simulink model "muscleLegs_task2"  (R2025b)
settings: Solver=ode23t  StartTime=0.0  StopTime=t_end  MaxStep=1e-3  RelTol=1e-4
values from neighbouring files (symbols this model uses):
  c = 0.05    [setup_muscleLegs_nm.m]
  CtrlPar = [tau_H_st; phi_K_tgt_st; P_K_st; D_K_st ... (first row only)    [setup_muscleLegs_ctrl.m]
  eref_se = 0.04    [setup_muscleLegs_nm.m]
  FmaxBFSH = 350    [setup_muscleLegs_nm.m]
  FmaxGLU = 4000    [setup_muscleLegs_nm.m]
  FmaxHFL = 2000    [setup_muscleLegs_nm.m]
  FmaxVAS = 5000    [setup_muscleLegs_nm.m]
  g = 9.81    [setup_muscleLegs_model.m]
  G_dtheta_GLU = 5    [setup_muscleLegs_ctrl.m]    (also in sim_muscleLegs_Task2.m = base_G_dtheta_GLU * optim_vals(15); sim_muscleLegs_Task3.m = base_G(2) * optim_vals(15))
  G_theta_GLU = 60    [setup_muscleLegs_ctrl.m]    (also in sim_muscleLegs_Task2.m = base_G_theta_GLU * optim_vals(14); sim_muscleLegs_Task3.m = base_G(1) * optim_vals(14))
  init_stim = 0.01    [setup_muscleLegs_nm.m]
  K = 5    [setup_muscleLegs_nm.m]
  l_HAT = 0.8    [setup_muscleLegs_model.m]
  l_shank = l_leg/2    (= 0.49)    [setup_muscleLegs_model.m]
  l_thigh = l_leg/2    (= 0.49)    [setup_muscleLegs_model.m]
  loptBFSH = 0.12    [setup_muscleLegs_nm.m]
  loptGLU = 0.11    [setup_muscleLegs_nm.m]
  loptHFL = 0.11    [setup_muscleLegs_nm.m]
  loptVAS = 0.08    [setup_muscleLegs_nm.m]
  lslackBFSH = 0.10    (= 0.1)    [setup_muscleLegs_nm.m]
  lslackGLU = 0.13    [setup_muscleLegs_nm.m]
  lslackHFL = 0.10    (= 0.1)    [setup_muscleLegs_nm.m]
  lslackVAS = 0.23    [setup_muscleLegs_nm.m]
  m_HAT = 54    [setup_muscleLegs_model.m]
  m_shank = 4    [setup_muscleLegs_model.m]
  m_thigh = 8    [setup_muscleLegs_model.m]
  N = 12    [cmaes_task1_2_set1.mat]    (also in cmaes_task1_2_set2.mat; cmaes_task2_2_set1.mat = 17; cmaes_task2_2_set2.mat = 17; cmaes_task3_crouch.mat = 17)
  phirefBFSH = 160*pi/180    (= 2.79252680319)    [setup_muscleLegs_nm.m]
  phirefGLU = 60*pi/180    (= 1.0471975512)    [setup_muscleLegs_nm.m]
  phirefHFL = 20*pi/180    (= 0.349065850399)    [setup_muscleLegs_nm.m]
  phirefVAS = 60*pi/180    (= 1.0471975512)    [setup_muscleLegs_nm.m]
  plane_height = 0.1    [setup_muscleLegs_model.m]
  plane_x = 100    [setup_muscleLegs_model.m]
  plane_z = 1    [setup_muscleLegs_model.m]
  r_foot = 0.01    [setup_muscleLegs_model.m]
  rBFSH = 0.04    [setup_muscleLegs_nm.m]
  rGLU = 0.08    [setup_muscleLegs_nm.m]
  rHFL = 0.08    [setup_muscleLegs_nm.m]
  rhoBFSH = 0.7    [setup_muscleLegs_nm.m]
  rhoGLU = 0.5    [setup_muscleLegs_nm.m]
  rhoHFL = 0.5    [setup_muscleLegs_nm.m]
  rhoVAS = 0.6    [setup_muscleLegs_nm.m]
  rVAS = 0.05    [setup_muscleLegs_nm.m]
  tau_act = 0.01    [setup_muscleLegs_nm.m]
  tau_deact = 0.04    [setup_muscleLegs_nm.m]
  theta_tgt = 0.001    [setup_muscleLegs_ctrl.m]    (also in sim_muscleLegs_Task2.m = 0 + (optim_vals(13) - 1) * 0.1; sim_muscleLegs_Task3.m = 0 + (optim_vals(13) - 1) * 0.1)
  vi_Ctrl_st = 1:4    [setup_muscleLegs_ctrl.m]
  vi_Ctrl_sw = 5:12    [setup_muscleLegs_ctrl.m]
  vmaxBFSH = 12    [setup_muscleLegs_nm.m]
  vmaxGLU = 12    [setup_muscleLegs_nm.m]
  vmaxHFL = 12    [setup_muscleLegs_nm.m]
  vmaxVAS = 12    [setup_muscleLegs_nm.m]
  w = 0.56    [setup_muscleLegs_nm.m]
  w_pe = w    (= 0.56)    [setup_muscleLegs_nm.m]
undefined symbols (not defined in the file or in its folder): l1, X, Y, Z
libraries: sm_lib x30, nesl_utility x19, simulink x1
(part 3 of 4)

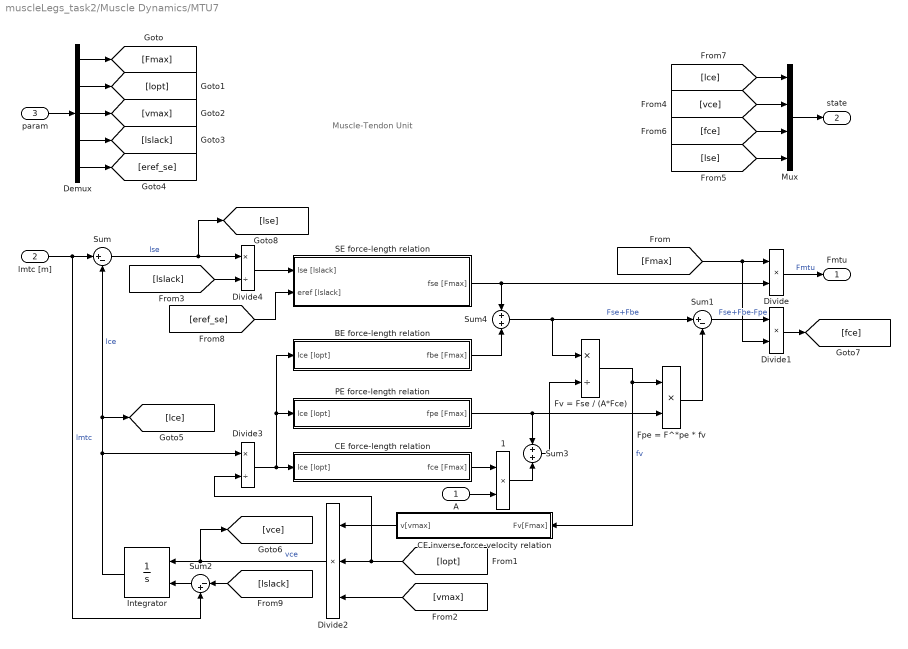
== system muscleLegs_task2/Muscle Dynamics/MTU7 ==
  note: Muscle-Tendon Unit
  A : Inport
  lmtc [m] : Inport  Port=2
  param : Inport  Port=3
  1 : Product  Inputs=**  InputSameDT=on  SaturateOnIntegerOverflow=on  OutDataTypeStr=Inherit: Same as first input
  BE force-length relation : Subsystem
  CE force-length relation : Subsystem
  CE inverse force-velocity relation : Subsystem
  Demux : Demux  Outputs=5
  Divide : Product
  Divide1 : Product
  Divide2 : Product  Inputs=3
  Divide3 : Product  Inputs=*/
  Divide4 : Product  Inputs=*/
  "Fpe = F^*pe * fv " : Product  InputSameDT=on  SaturateOnIntegerOverflow=on  OutDataTypeStr=Inherit: Same as first input
  Fv = Fse / (A*Fce) : Product  Inputs=*/  InputSameDT=on  SaturateOnIntegerOverflow=on  OutDataTypeStr=Inherit: Same as first input
  Integrator : Integrator  InitialConditionSource=external  LowerSaturationLimit=0.05
  Mux : Mux
  PE force-length relation : Subsystem
  SE force-length relation : Subsystem
  Sum : Sum  Inputs=|+-  InputSameDT=on  SaturateOnIntegerOverflow=on  OutDataTypeStr=Inherit: Same as first input
  Sum1 : Sum  Inputs=|+-  InputSameDT=on  SaturateOnIntegerOverflow=on  OutDataTypeStr=Inherit: Same as first input
  Sum2 : Sum  Inputs=|-+  InputSameDT=on  SaturateOnIntegerOverflow=on  OutDataTypeStr=Inherit: Same as first input
  Sum3 : Sum  InputSameDT=on  SaturateOnIntegerOverflow=on  OutDataTypeStr=Inherit: Same as first input
  Sum4 : Sum  InputSameDT=on  SaturateOnIntegerOverflow=on  OutDataTypeStr=Inherit: Same as first input
  Fmtu : Outport  InitialOutput=0  VectorParamsAs1DForOutWhenUnconnected=off
  state : Outport  Port=2  InitialOutput=0  VectorParamsAs1DForOutWhenUnconnected=off
  wires:
  Integrator/1 -> Divide3/1, [lce], Sum/2  "lce"
  Divide3/1 -> CE force-length relation/1(lce [lopt]), PE force-length relation/1(lce [lopt]), BE force-length relation/1(lce [lopt])
  Fv = Fse / (A*Fce)/1 -> CE inverse force-velocity relation/1(Fv[Fmax]), "Fpe = F^*pe * fv "/1  "fv"
  Divide2/1 -> [vce], Integrator/1  "vce"
  lmtc [m]/1 -> Sum/1, Sum2/2  "lmtc"
  Divide/1 -> Fmtu/1  "Fmtu"
  Divide4/1 -> SE force-length relation/1(lse [lslack])
  SE force-length relation/1(fse [Fmax]) -> Sum4/1, Divide/2
  Sum2/1 -> Integrator/2
  [lslack] -> Sum2/1
  CE force-length relation/1(fce [Fmax]) -> 1/1
  PE force-length relation/1(fpe [Fmax]) -> "Fpe = F^*pe * fv "/2, Sum3/1
  1/1 -> Sum3/2
  BE force-length relation/1(fbe [Fmax]) -> Sum4/2
  Sum3/1 -> Fv = Fse / (A*Fce)/2
  CE inverse force-velocity relation/1(v[vmax]) -> Divide2/1
  A/1 -> 1/2
  Sum4/1 -> Sum1/1, Fv = Fse / (A*Fce)/1  "Fse+Fbe"
  "Fpe = F^*pe * fv "/1 -> Sum1/2
  Sum1/1 -> Divide1/1  "Fse+Fbe-Fpe"
  Divide1/1 -> [fce]
  Sum/1 -> [lse], Divide4/1  "lse"
  [lopt] -> Divide2/2, Divide3/2
  [vmax] -> Divide2/3
  [lslack] -> Divide4/2
  param/1 -> Demux/1
  Demux/1 -> [Fmax]
  Demux/2 -> [lopt]
  Demux/4 -> [lslack]
  Demux/3 -> [vmax]
  Demux/5 -> [eref_se]
  [Fmax] -> Divide1/2, Divide/1
  Mux/1 -> state/1
  [lce] -> Mux/1
  [vce] -> Mux/2
  [fce] -> Mux/3
  [lse] -> Mux/4
  [eref_se] -> SE force-length relation/2(eref [lslack])

== system muscleLegs_task2/Neural Control/Stance L ==
  CtrlPar : Inport
  phi_K : Inport  Port=2
  d_phi_K : Inport  Port=3
  d_theta : Inport  Port=4
  theta : Inport  Port=5
  d_theta1 : Inport  Port=6
  theta1 : Inport  Port=7
  Enable : EnablePort
  Constant : Constant  Value=theta_tgt
  Constant1 : Constant  Value=theta_tgt
  Constant2 : Constant  Value=0
  Demux : Demux  Outputs=length(vi_Ctrl_st)
  Divide : Product
  Divide1 : Product
  Gain : Gain  Gain=-1
  Gain1 : Gain  Gain=G_theta_GLU
  Gain2 : Gain  Gain=G_dtheta_GLU
  Gain3 : Gain  Gain=-G_theta_GLU
  Gain4 : Gain  Gain=-G_dtheta_GLU
  Sum{,1,5..6} (4 alike) : Sum  Inputs=|+-
  Sum2 : Sum  Inputs=|++
  Sum3 : Sum  Inputs=|++
  Sum4 : Sum  Inputs=|++
  extension : Saturate  UpperLimit=1  LowerLimit=0.01
  extension1 : Saturate  UpperLimit=1  LowerLimit=0.01
  flexion : Saturate  UpperLimit=1  LowerLimit=0.01
  flexion1 : Saturate  UpperLimit=1  LowerLimit=0.01
  S_VAS : Outport  OutputWhenDisabled=reset  InitialOutput=0
  S_BFSH : Outport  Port=2  OutputWhenDisabled=reset  InitialOutput=0
  S_GLU : Outport  Port=3  OutputWhenDisabled=reset  InitialOutput=0
  S_HFL : Outport  Port=4  OutputWhenDisabled=reset  InitialOutput=0
  wires:
  Divide1/1 -> Sum2/2
  d_phi_K/1 -> Sum1/2
  phi_K/1 -> Sum/2
  Divide/1 -> Sum2/1
  Sum/1 -> Divide/2
  Sum1/1 -> Divide1/2
  Constant2/1 -> Sum1/1
  CtrlPar/1 -> Demux/1
  Demux/2 -> Sum/1  "phi_K_tgt_st"
  Demux/3 -> Divide/1  "P_K_st"
  Demux/4 -> Divide1/1  "D_K_st"
  extension/1 -> S_VAS/1
  Gain/1 -> extension/1
  Sum2/1 -> flexion/1, Gain/1
  flexion/1 -> S_BFSH/1
  Sum3/1 -> extension1/1
  extension1/1 -> S_GLU/1
  flexion1/1 -> S_HFL/1
  Gain1/1 -> Sum3/1
  Gain2/1 -> Sum3/2
  d_theta/1 -> Gain2/1
  d_theta1/1 -> Gain4/1
  Sum4/1 -> flexion1/1
  Gain4/1 -> Sum4/2
  Gain3/1 -> Sum4/1
  theta/1 -> Sum5/1
  Sum5/1 -> Gain1/1
  Constant/1 -> Sum5/2
  theta1/1 -> Sum6/1
  Sum6/1 -> Gain3/1
  Constant1/1 -> Sum6/2

== system muscleLegs_task2/Neural Control/Stance R ==
  CtrlPar : Inport
  phi_K : Inport  Port=2
  d_phi_K : Inport  Port=3
  d_theta1 : Inport  Port=4
  theta1 : Inport  Port=5
  d_theta2 : Inport  Port=6
  theta2 : Inport  Port=7
  Enable : EnablePort
  Constant : Constant  Value=theta_tgt
  Constant1 : Constant  Value=theta_tgt
  Constant2 : Constant  Value=0
  Demux : Demux  Outputs=length(vi_Ctrl_st)
  Divide : Product
  Divide1 : Product
  Gain : Gain  Gain=-1
  Gain1 : Gain  Gain=G_theta_GLU
  Gain2 : Gain  Gain=G_dtheta_GLU
  Gain3 : Gain  Gain=-G_theta_GLU
  Gain4 : Gain  Gain=-G_dtheta_GLU
  Sum{,1,5..6} (4 alike) : Sum  Inputs=|+-
  Sum2 : Sum  Inputs=|++
  Sum3 : Sum  Inputs=|++
  Sum4 : Sum  Inputs=|++
  extension : Saturate  UpperLimit=1  LowerLimit=0.01
  extension1 : Saturate  UpperLimit=1  LowerLimit=0.01
  flexion : Saturate  UpperLimit=1  LowerLimit=0.01
  flexion1 : Saturate  UpperLimit=1  LowerLimit=0.01
  S_VAS : Outport  OutputWhenDisabled=reset  InitialOutput=0
  S_BFSH : Outport  Port=2  OutputWhenDisabled=reset  InitialOutput=0
  S_GLU : Outport  Port=3  OutputWhenDisabled=reset  InitialOutput=0
  S_HFL : Outport  Port=4  OutputWhenDisabled=reset  InitialOutput=0
  wires:
  Divide1/1 -> Sum2/2
  d_phi_K/1 -> Sum1/2
  phi_K/1 -> Sum/2
  Divide/1 -> Sum2/1
  Sum/1 -> Divide/2
  Sum1/1 -> Divide1/2
  Constant2/1 -> Sum1/1
  CtrlPar/1 -> Demux/1
  Demux/2 -> Sum/1  "phi_K_tgt_st"
  Demux/3 -> Divide/1  "P_K_st"
  Demux/4 -> Divide1/1  "D_K_st"
  flexion/1 -> S_BFSH/1
  Sum2/1 -> flexion/1, Gain/1
  extension/1 -> S_VAS/1
  Gain/1 -> extension/1
  Sum4/1 -> flexion1/1
  Gain3/1 -> Sum4/1
  Gain4/1 -> Sum4/2
  d_theta2/1 -> Gain4/1
  Sum3/1 -> extension1/1
  Gain2/1 -> Sum3/2
  extension1/1 -> S_GLU/1
  flexion1/1 -> S_HFL/1
  Gain1/1 -> Sum3/1
  theta1/1 -> Sum5/1
  Sum5/1 -> Gain1/1
  d_theta1/1 -> Gain2/1
  theta2/1 -> Sum6/1
  Sum6/1 -> Gain3/1
  Constant/1 -> Sum5/2
  Constant1/1 -> Sum6/2

== system muscleLegs_task2/Neural Control/Swing L ==
  CtrlPar : Inport
  phi_H : Inport  Port=2
  d_phi_H : Inport  Port=3
  phi_K : Inport  Port=4
  d_phi_K : Inport  Port=5
  Enable : EnablePort
  Constant2 : Constant  Value=0
  Constant3 : Constant  Value=0
  Demux1 : Demux  Outputs=length(vi_Ctrl_sw)
  Divide{,1..3} (4 alike) : Product
  Gain : Gain  Gain=-1
  Gain1 : Gain  Gain=-1
  Gain4 : Gain  Gain=180/pi
  Gain5 : Gain  Gain=180/pi
  Multiport Switch : MultiPortSwitch  DataPortOrder=Zero-based contiguous  Inputs=2  zeroidx=on  SaturateOnIntegerOverflow=off  InputSameDT=off
  Mux4 : Mux  Inputs=2
  Relational Operator : RelationalOperator  Operator=>  OutDataTypeStr=boolean  RndMeth=Simplest  InputSameDT=off
  Scope1 : Scope  NumInputPorts=3
      settings: ActiveDisplayYMinimum=-0.56332  ActiveDisplayYMaximum=0.70659  DataLoggingVariableName=ScopeData2
  Sum{,1,3..4} (4 alike) : Sum  Inputs=|+-
  Sum2 : Sum  Inputs=|++
  Sum5 : Sum  Inputs=|++
  extension : Saturate  UpperLimit=1  LowerLimit=0.01
  extension1 : Saturate  UpperLimit=1  LowerLimit=0.01
  flexion : Saturate  UpperLimit=1  LowerLimit=0.01
  flexion1 : Saturate  UpperLimit=1  LowerLimit=0.01
  phi_L : Fcn  Expr=u(1) - 0.5*u(2)
  S_VAS : Outport  OutputWhenDisabled=reset  InitialOutput=0
  S_BFSH : Outport  Port=2  OutputWhenDisabled=reset  InitialOutput=0
  S_GLU : Outport  Port=3  OutputWhenDisabled=reset  InitialOutput=0
  S_HFL : Outport  Port=4  OutputWhenDisabled=reset  InitialOutput=0
  wires:
  Sum1/1 -> Divide1/2
  Sum/1 -> Divide/2
  Divide1/1 -> Sum2/2
  Constant3/1 -> Sum1/1
  Divide/1 -> Sum2/1
  d_phi_H/1 -> Sum1/2
  Mux4/1 -> phi_L/1
  phi_H/1 -> Mux4/1
  phi_L/1 -> Relational Operator/1, Sum/2, Gain4/1
  Multiport Switch/1 -> Sum3/1, Gain5/1  "phi_K_tgt_sw"
  phi_K/1 -> Sum3/2, Mux4/2
  Divide3/1 -> Sum5/2
  Constant2/1 -> Sum4/1
  Sum4/1 -> Divide3/2
  Divide2/1 -> Sum5/1
  Sum3/1 -> Divide2/2
  d_phi_K/1 -> Sum4/2
  Relational Operator/1 -> Multiport Switch/1, Scope1/2
  Gain4/1 -> Scope1/1
  Gain5/1 -> Scope1/3
  Demux1/1 -> Sum/1  "phi_H_tgt_sw"
  CtrlPar/1 -> Demux1/1
  Demux1/2 -> Divide/1  "P_H_sw"
  Demux1/3 -> Divide1/1  "D_H_sw"
  Demux1/4 -> Multiport Switch/2  "v_phi_K_tgt_sw(1)"
  Demux1/5 -> Multiport Switch/3  "v_phi_K_tgt_sw(2)"
  Demux1/7 -> Divide2/1  "P_K_sw"
  Demux1/8 -> Divide3/1  "D_K_sw"
  Demux1/6 -> Relational Operator/2  "phi_H_ref_sw"
  Sum5/1 -> flexion/1, Gain/1
  Gain/1 -> extension/1
  extension/1 -> S_VAS/1
  flexion/1 -> S_BFSH/1
  Sum2/1 -> Gain1/1, flexion1/1  "tau_H_st"
  Gain1/1 -> extension1/1
  flexion1/1 -> S_HFL/1
  extension1/1 -> S_GLU/1

== system muscleLegs_task2/Neural Control/Swing R ==
  CtrlPar : Inport
  phi_H : Inport  Port=2
  d_phi_H : Inport  Port=3
  phi_K : Inport  Port=4
  d_phi_K : Inport  Port=5
  Enable : EnablePort
  Constant2 : Constant  Value=0
  Constant3 : Constant  Value=0
  Demux1 : Demux  Outputs=length(vi_Ctrl_sw)
  Divide{,1..3} (4 alike) : Product
  Gain : Gain  Gain=-1
  Gain1 : Gain  Gain=-1
  Gain4 : Gain  Gain=180/pi
  Gain5 : Gain  Gain=180/pi
  Multiport Switch : MultiPortSwitch  DataPortOrder=Zero-based contiguous  Inputs=2  zeroidx=on  SaturateOnIntegerOverflow=off  InputSameDT=off
  Mux4 : Mux  Inputs=2
  Relational Operator : RelationalOperator  Operator=>  OutDataTypeStr=boolean  RndMeth=Simplest  InputSameDT=off
  Scope1 : Scope  NumInputPorts=3
      settings: ActiveDisplayYMinimum=-0.56332  ActiveDisplayYMaximum=0.70659  DataLoggingVariableName=ScopeData2
  Sum{,1,3..4} (4 alike) : Sum  Inputs=|+-
  Sum2 : Sum  Inputs=|++
  Sum5 : Sum  Inputs=|++
  extension : Saturate  UpperLimit=1  LowerLimit=0.01
  extension1 : Saturate  UpperLimit=1  LowerLimit=0.01
  flexion : Saturate  UpperLimit=1  LowerLimit=0.01
  flexion1 : Saturate  UpperLimit=1  LowerLimit=0.01
  phi_L : Fcn  Expr=u(1) - 0.5*u(2)
  S_VAS : Outport  OutputWhenDisabled=reset  InitialOutput=0
  S_BFSH : Outport  Port=2  OutputWhenDisabled=reset  InitialOutput=0
  S_GLU : Outport  Port=3  OutputWhenDisabled=reset  InitialOutput=0
  S_HFL : Outport  Port=4  OutputWhenDisabled=reset  InitialOutput=0
  wires:
  Sum1/1 -> Divide1/2
  Sum/1 -> Divide/2
  Divide1/1 -> Sum2/2
  Constant3/1 -> Sum1/1
  Divide/1 -> Sum2/1
  d_phi_H/1 -> Sum1/2
  Mux4/1 -> phi_L/1
  phi_H/1 -> Mux4/1
  phi_L/1 -> Relational Operator/1, Sum/2, Gain4/1
  Multiport Switch/1 -> Sum3/1, Gain5/1  "phi_K_tgt_sw"
  phi_K/1 -> Sum3/2, Mux4/2
  Divide3/1 -> Sum5/2
  Constant2/1 -> Sum4/1
  Sum4/1 -> Divide3/2
  Divide2/1 -> Sum5/1
  Sum3/1 -> Divide2/2
  d_phi_K/1 -> Sum4/2
  Relational Operator/1 -> Multiport Switch/1, Scope1/2
  Gain4/1 -> Scope1/1
  Gain5/1 -> Scope1/3
  Demux1/1 -> Sum/1  "phi_H_tgt_sw"
  CtrlPar/1 -> Demux1/1
  Demux1/2 -> Divide/1  "P_H_sw"
  Demux1/3 -> Divide1/1  "D_H_sw"
  Demux1/4 -> Multiport Switch/2  "v_phi_K_tgt_sw(1)"
  Demux1/5 -> Multiport Switch/3  "v_phi_K_tgt_sw(2)"
  Demux1/7 -> Divide2/1  "P_K_sw"
  Demux1/8 -> Divide3/1  "D_K_sw"
  Demux1/6 -> Relational Operator/2  "phi_H_ref_sw"
  Sum5/1 -> flexion/1, Gain/1
  Gain/1 -> extension/1
  extension/1 -> S_VAS/1
  flexion/1 -> S_BFSH/1
  Sum2/1 -> flexion1/1, Gain1/1  "tau_H_st"
  Gain1/1 -> extension1/1
  extension1/1 -> S_GLU/1
  flexion1/1 -> S_HFL/1

== system muscleLegs_task2/Muscle Dynamics/MTU/BE force-length relation ==
  note: Buffer Elasticity BE
  lce [lopt] : Inport
  Constant1 : Constant  Value=1-w
  Math Function : Math  Operator=square  SignedPower=on
  Mux1 : Mux  Inputs=2
  Sum4 : Sum  Inputs=|+-  InputSameDT=on  SaturateOnIntegerOverflow=on  OutDataTypeStr=Inherit: Same as first input
  force above slack length : Fcn  Expr=u(2)*(u(1)<0)
  reference strain [lslack] : Constant  Value=w/2
  relative strain : Product  Inputs=*/
  fbe [Fmax] : Outport  VectorParamsAs1DForOutWhenUnconnected=off
  wires:
  lce [lopt]/1 -> Sum4/1
  Mux1/1 -> force above slack length/1
  force above slack length/1 -> fbe [Fmax]/1
  Math Function/1 -> Mux1/2
  relative strain/1 -> Math Function/1
  reference strain [lslack]/1 -> relative strain/2
  Sum4/1 -> relative strain/1, Mux1/1
  Constant1/1 -> Sum4/2

== system muscleLegs_task2/Muscle Dynamics/MTU/CE force-length relation ==
  note: CE Force-Length Relationship
  lce [lopt] : Inport
  Abs : Abs  SaturateOnIntegerOverflow=off
  Constant1 : Constant
  Constant2 : Constant  Value=3
  Gain : Gain  Gain=log(c)
  Math Function : Math  SignedPower=on
  Math Function1 : Math  Operator=pow  SignedPower=on
  Sum4 : Sum  Inputs=|+-  InputSameDT=on  SaturateOnIntegerOverflow=on  OutDataTypeStr=Inherit: Same as first input
  normalized position : Product  Inputs=*/
  relative width : Constant  Value=w
  fce [Fmax] : Outport  VectorParamsAs1DForOutWhenUnconnected=off
  wires:
  lce [lopt]/1 -> Sum4/1
  relative width/1 -> normalized position/2
  Constant1/1 -> Sum4/2
  Sum4/1 -> Abs/1
  Abs/1 -> normalized position/1
  normalized position/1 -> Math Function1/1
  Constant2/1 -> Math Function1/2
  Math Function1/1 -> Gain/1
  Gain/1 -> Math Function/1
  Math Function/1 -> fce [Fmax]/1

== system muscleLegs_task2/Muscle Dynamics/MTU/CE inverse force-velocity relation ==
  note: CE Inverse Force-Velocity Relationship
  Fv[Fmax] : Inport
  1 : Product  Inputs=/*
  Constant{1,3..4,8} (4 alike) : Constant
  Constant2 : Constant  Value=N
  Constant5 : Constant  Value=N
  Curvature : Gain  Gain=K  SaturateOnIntegerOverflow=on  OutDataTypeStr=Inherit: Same as input  ParamDataTypeStr=Inherit: Same as input
  Curvature1 : Gain  Gain=7.56*K  SaturateOnIntegerOverflow=on  OutDataTypeStr=Inherit: Same as input  ParamDataTypeStr=Inherit: Same as input
  Mux : Mux  Inputs=2
  Mux1 : Mux  Inputs=3
  Mux2 : Mux  Inputs=3
  Slope : Gain  Gain=1e-2  SaturateOnIntegerOverflow=on  OutDataTypeStr=Inherit: Same as input  ParamDataTypeStr=Inherit: Same as input
  Sum1 : Sum  Inputs=|++  InputSameDT=on  SaturateOnIntegerOverflow=on  OutDataTypeStr=Inherit: Same as first input
  Sum2 : Sum  InputSameDT=on  SaturateOnIntegerOverflow=on  OutDataTypeStr=Inherit: Same as first input
  Sum3 : Sum  Inputs=++|  InputSameDT=on  SaturateOnIntegerOverflow=on  OutDataTypeStr=Inherit: Same as first input
  Sum4 : Sum  Inputs=|+-  InputSameDT=on  SaturateOnIntegerOverflow=on  OutDataTypeStr=Inherit: Same as first input
  Sum5 : Sum  Inputs=|-+  InputSameDT=on  SaturateOnIntegerOverflow=on  OutDataTypeStr=Inherit: Same as first input
  Sum6 : Sum  Inputs=-+|  InputSameDT=on  SaturateOnIntegerOverflow=on  OutDataTypeStr=Inherit: Same as first input
  Sum7 : Sum  Inputs=|++  InputSameDT=on  SaturateOnIntegerOverflow=on  OutDataTypeStr=Inherit: Same as first input
  Sum8 : Sum  Inputs=+-|  InputSameDT=on  SaturateOnIntegerOverflow=on  OutDataTypeStr=Inherit: Same as first input
  Sum9 : Sum  InputSameDT=on  SaturateOnIntegerOverflow=on  OutDataTypeStr=Inherit: Same as first input
  concentric branch : Fcn  Expr=u(1) * (u(2)<=1)
  excentric branch : Fcn  Expr=u(2) * (u(1)>1)*(u(1)<=u(3))
  excentric overshoot : Fcn  Expr=u(3) * (u(2)>u(1))
  v_concentric : Product  Inputs=*/
  v_excentric <N : Product  Inputs=*/
  v[vmax] : Outport  VectorParamsAs1DForOutWhenUnconnected=off
  wires:
  Curvature/1 -> Sum3/2
  Constant1/1 -> Sum4/2, Sum3/1
  Sum4/1 -> v_concentric/1
  Sum3/1 -> v_concentric/2
  1/1 -> Sum7/1, Curvature1/1
  Constant4/1 -> Sum7/2, Sum8/1
  Curvature1/1 -> Sum8/2
  Sum8/1 -> v_excentric <N/2
  Sum7/1 -> v_excentric <N/1
  v_concentric/1 -> Mux/1
  Fv[Fmax]/1 -> Sum4/1, Curvature/1, Sum6/2, Mux/2, Mux1/1, Mux2/2
  Sum9/1 -> v[vmax]/1
  Sum2/1 -> Sum9/2
  excentric overshoot/1 -> Sum2/2
  Slope/1 -> Sum1/1
  Constant8/1 -> Sum1/2
  Sum6/1 -> 1/2, Slope/1
  Constant2/1 -> Sum6/1, Sum5/2
  Sum5/1 -> 1/1
  Constant3/1 -> Sum5/1
  Mux/1 -> concentric branch/1
  Mux1/1 -> excentric branch/1
  v_excentric <N/1 -> Mux1/2
  Mux2/1 -> excentric overshoot/1
  concentric branch/1 -> Sum9/1
  excentric branch/1 -> Sum2/1
  Constant5/1 -> Mux1/3, Mux2/1
  Sum1/1 -> Mux2/3

== system muscleLegs_task2/Muscle Dynamics/MTU/PE force-length relation ==
  note: Parallel Elasticity PE
  lce [lopt] : Inport
  Constant3 : Constant
  Math Function2 : Math  Operator=square  SignedPower=on
  Mux : Mux  Inputs=2
  Sum1 : Sum  Inputs=|+-  InputSameDT=on  SaturateOnIntegerOverflow=on  OutDataTypeStr=Inherit: Same as first input
  force above slack length : Fcn  Expr=u(2) * (u(1)>1)
  reference strain [lopt] : Constant  Value=w_pe
  relative strain : Product  Inputs=*/
  fpe [Fmax] : Outport  VectorParamsAs1DForOutWhenUnconnected=off
  wires:
  Mux/1 -> force above slack length/1
  lce [lopt]/1 -> Mux/1, Sum1/1
  Constant3/1 -> Sum1/2
  Sum1/1 -> relative strain/1
  reference strain [lopt]/1 -> relative strain/2
  relative strain/1 -> Math Function2/1
  Math Function2/1 -> Mux/2
  force above slack length/1 -> fpe [Fmax]/1

== system muscleLegs_task2/Muscle Dynamics/MTU/SE force-length relation ==
  note: SE Force-Length Relationship
  lse [lslack] : Inport
  eref [lslack] : Inport  Port=2
  Constant1 : Constant
  Math Function : Math  Operator=square  SignedPower=on
  Mux : Mux  Inputs=2
  Sum4 : Sum  Inputs=|+-  InputSameDT=on  SaturateOnIntegerOverflow=on  OutDataTypeStr=Inherit: Same as first input
  force above slack length : Fcn  Expr=u(2)*(u(1)>1)
  relative strain : Product  Inputs=*/
  fse [Fmax] : Outport  VectorParamsAs1DForOutWhenUnconnected=off
  wires:
  Mux/1 -> force above slack length/1
  force above slack length/1 -> fse [Fmax]/1
  Math Function/1 -> Mux/2
  lse [lslack]/1 -> Mux/1, Sum4/1
  relative strain/1 -> Math Function/1
  eref [lslack]/1 -> relative strain/2
  Sum4/1 -> relative strain/1
  Constant1/1 -> Sum4/2

== system muscleLegs_task2/Muscle Dynamics/MTU1/BE force-length relation ==
  note: Buffer Elasticity BE
  lce [lopt] : Inport
  Constant1 : Constant  Value=1-w
  Math Function : Math  Operator=square  SignedPower=on
  Mux1 : Mux  Inputs=2
  Sum4 : Sum  Inputs=|+-  InputSameDT=on  SaturateOnIntegerOverflow=on  OutDataTypeStr=Inherit: Same as first input
  force above slack length : Fcn  Expr=u(2)*(u(1)<0)
  reference strain [lslack] : Constant  Value=w/2
  relative strain : Product  Inputs=*/
  fbe [Fmax] : Outport  VectorParamsAs1DForOutWhenUnconnected=off
  wires:
  lce [lopt]/1 -> Sum4/1
  Mux1/1 -> force above slack length/1
  force above slack length/1 -> fbe [Fmax]/1
  Math Function/1 -> Mux1/2
  relative strain/1 -> Math Function/1
  reference strain [lslack]/1 -> relative strain/2
  Sum4/1 -> relative strain/1, Mux1/1
  Constant1/1 -> Sum4/2

== system muscleLegs_task2/Muscle Dynamics/MTU1/CE force-length relation ==
  note: CE Force-Length Relationship
  lce [lopt] : Inport
  Abs : Abs  SaturateOnIntegerOverflow=off
  Constant1 : Constant
  Constant2 : Constant  Value=3
  Gain : Gain  Gain=log(c)
  Math Function : Math  SignedPower=on
  Math Function1 : Math  Operator=pow  SignedPower=on
  Sum4 : Sum  Inputs=|+-  InputSameDT=on  SaturateOnIntegerOverflow=on  OutDataTypeStr=Inherit: Same as first input
  normalized position : Product  Inputs=*/
  relative width : Constant  Value=w
  fce [Fmax] : Outport  VectorParamsAs1DForOutWhenUnconnected=off
  wires:
  lce [lopt]/1 -> Sum4/1
  relative width/1 -> normalized position/2
  Constant1/1 -> Sum4/2
  Sum4/1 -> Abs/1
  Abs/1 -> normalized position/1
  normalized position/1 -> Math Function1/1
  Constant2/1 -> Math Function1/2
  Math Function1/1 -> Gain/1
  Gain/1 -> Math Function/1
  Math Function/1 -> fce [Fmax]/1

== system muscleLegs_task2/Muscle Dynamics/MTU1/CE inverse force-velocity relation ==
  note: CE Inverse Force-Velocity Relationship
  Fv[Fmax] : Inport
  1 : Product  Inputs=/*
  Constant{1,3..4,8} (4 alike) : Constant
  Constant2 : Constant  Value=N
  Constant5 : Constant  Value=N
  Curvature : Gain  Gain=K  SaturateOnIntegerOverflow=on  OutDataTypeStr=Inherit: Same as input  ParamDataTypeStr=Inherit: Same as input
  Curvature1 : Gain  Gain=7.56*K  SaturateOnIntegerOverflow=on  OutDataTypeStr=Inherit: Same as input  ParamDataTypeStr=Inherit: Same as input
  Mux : Mux  Inputs=2
  Mux1 : Mux  Inputs=3
  Mux2 : Mux  Inputs=3
  Slope : Gain  Gain=1e-2  SaturateOnIntegerOverflow=on  OutDataTypeStr=Inherit: Same as input  ParamDataTypeStr=Inherit: Same as input
  Sum1 : Sum  Inputs=|++  InputSameDT=on  SaturateOnIntegerOverflow=on  OutDataTypeStr=Inherit: Same as first input
  Sum2 : Sum  InputSameDT=on  SaturateOnIntegerOverflow=on  OutDataTypeStr=Inherit: Same as first input
  Sum3 : Sum  Inputs=++|  InputSameDT=on  SaturateOnIntegerOverflow=on  OutDataTypeStr=Inherit: Same as first input
  Sum4 : Sum  Inputs=|+-  InputSameDT=on  SaturateOnIntegerOverflow=on  OutDataTypeStr=Inherit: Same as first input
  Sum5 : Sum  Inputs=|-+  InputSameDT=on  SaturateOnIntegerOverflow=on  OutDataTypeStr=Inherit: Same as first input
  Sum6 : Sum  Inputs=-+|  InputSameDT=on  SaturateOnIntegerOverflow=on  OutDataTypeStr=Inherit: Same as first input
  Sum7 : Sum  Inputs=|++  InputSameDT=on  SaturateOnIntegerOverflow=on  OutDataTypeStr=Inherit: Same as first input
  Sum8 : Sum  Inputs=+-|  InputSameDT=on  SaturateOnIntegerOverflow=on  OutDataTypeStr=Inherit: Same as first input
  Sum9 : Sum  InputSameDT=on  SaturateOnIntegerOverflow=on  OutDataTypeStr=Inherit: Same as first input
  concentric branch : Fcn  Expr=u(1) * (u(2)<=1)
  excentric branch : Fcn  Expr=u(2) * (u(1)>1)*(u(1)<=u(3))
  excentric overshoot : Fcn  Expr=u(3) * (u(2)>u(1))
  v_concentric : Product  Inputs=*/
  v_excentric <N : Product  Inputs=*/
  v[vmax] : Outport  VectorParamsAs1DForOutWhenUnconnected=off
  wires:
  Curvature/1 -> Sum3/2
  Constant1/1 -> Sum4/2, Sum3/1
  Sum4/1 -> v_concentric/1
  Sum3/1 -> v_concentric/2
  1/1 -> Sum7/1, Curvature1/1
  Constant4/1 -> Sum7/2, Sum8/1
  Curvature1/1 -> Sum8/2
  Sum8/1 -> v_excentric <N/2
  Sum7/1 -> v_excentric <N/1
  v_concentric/1 -> Mux/1
  Fv[Fmax]/1 -> Sum4/1, Curvature/1, Sum6/2, Mux/2, Mux1/1, Mux2/2
  Sum9/1 -> v[vmax]/1
  Sum2/1 -> Sum9/2
  excentric overshoot/1 -> Sum2/2
  Slope/1 -> Sum1/1
  Constant8/1 -> Sum1/2
  Sum6/1 -> 1/2, Slope/1
  Constant2/1 -> Sum6/1, Sum5/2
  Sum5/1 -> 1/1
  Constant3/1 -> Sum5/1
  Mux/1 -> concentric branch/1
  Mux1/1 -> excentric branch/1
  v_excentric <N/1 -> Mux1/2
  Mux2/1 -> excentric overshoot/1
  concentric branch/1 -> Sum9/1
  excentric branch/1 -> Sum2/1
  Constant5/1 -> Mux1/3, Mux2/1
  Sum1/1 -> Mux2/3

== system muscleLegs_task2/Muscle Dynamics/MTU1/PE force-length relation ==
  note: Parallel Elasticity PE
  lce [lopt] : Inport
  Constant3 : Constant
  Math Function2 : Math  Operator=square  SignedPower=on
  Mux : Mux  Inputs=2
  Sum1 : Sum  Inputs=|+-  InputSameDT=on  SaturateOnIntegerOverflow=on  OutDataTypeStr=Inherit: Same as first input
  force above slack length : Fcn  Expr=u(2) * (u(1)>1)
  reference strain [lopt] : Constant  Value=w_pe
  relative strain : Product  Inputs=*/
  fpe [Fmax] : Outport  VectorParamsAs1DForOutWhenUnconnected=off
  wires:
  Mux/1 -> force above slack length/1
  lce [lopt]/1 -> Mux/1, Sum1/1
  Constant3/1 -> Sum1/2
  Sum1/1 -> relative strain/1
  reference strain [lopt]/1 -> relative strain/2
  relative strain/1 -> Math Function2/1
  Math Function2/1 -> Mux/2
  force above slack length/1 -> fpe [Fmax]/1

== system muscleLegs_task2/Muscle Dynamics/MTU1/SE force-length relation ==
  note: SE Force-Length Relationship
  lse [lslack] : Inport
  eref [lslack] : Inport  Port=2
  Constant1 : Constant
  Math Function : Math  Operator=square  SignedPower=on
  Mux : Mux  Inputs=2
  Sum4 : Sum  Inputs=|+-  InputSameDT=on  SaturateOnIntegerOverflow=on  OutDataTypeStr=Inherit: Same as first input
  force above slack length : Fcn  Expr=u(2)*(u(1)>1)
  relative strain : Product  Inputs=*/
  fse [Fmax] : Outport  VectorParamsAs1DForOutWhenUnconnected=off
  wires:
  Mux/1 -> force above slack length/1
  force above slack length/1 -> fse [Fmax]/1
  Math Function/1 -> Mux/2
  lse [lslack]/1 -> Mux/1, Sum4/1
  relative strain/1 -> Math Function/1
  eref [lslack]/1 -> relative strain/2
  Sum4/1 -> relative strain/1
  Constant1/1 -> Sum4/2

== system muscleLegs_task2/Muscle Dynamics/MTU2/BE force-length relation ==
  note: Buffer Elasticity BE
  lce [lopt] : Inport
  Constant1 : Constant  Value=1-w
  Math Function : Math  Operator=square  SignedPower=on
  Mux1 : Mux  Inputs=2
  Sum4 : Sum  Inputs=|+-  InputSameDT=on  SaturateOnIntegerOverflow=on  OutDataTypeStr=Inherit: Same as first input
  force above slack length : Fcn  Expr=u(2)*(u(1)<0)
  reference strain [lslack] : Constant  Value=w/2
  relative strain : Product  Inputs=*/
  fbe [Fmax] : Outport  VectorParamsAs1DForOutWhenUnconnected=off
  wires:
  lce [lopt]/1 -> Sum4/1
  Mux1/1 -> force above slack length/1
  force above slack length/1 -> fbe [Fmax]/1
  Math Function/1 -> Mux1/2
  relative strain/1 -> Math Function/1
  reference strain [lslack]/1 -> relative strain/2
  Sum4/1 -> relative strain/1, Mux1/1
  Constant1/1 -> Sum4/2

== system muscleLegs_task2/Muscle Dynamics/MTU2/CE force-length relation ==
  note: CE Force-Length Relationship
  lce [lopt] : Inport
  Abs : Abs  SaturateOnIntegerOverflow=off
  Constant1 : Constant
  Constant2 : Constant  Value=3
  Gain : Gain  Gain=log(c)
  Math Function : Math  SignedPower=on
  Math Function1 : Math  Operator=pow  SignedPower=on
  Sum4 : Sum  Inputs=|+-  InputSameDT=on  SaturateOnIntegerOverflow=on  OutDataTypeStr=Inherit: Same as first input
  normalized position : Product  Inputs=*/
  relative width : Constant  Value=w
  fce [Fmax] : Outport  VectorParamsAs1DForOutWhenUnconnected=off
  wires:
  lce [lopt]/1 -> Sum4/1
  relative width/1 -> normalized position/2
  Constant1/1 -> Sum4/2
  Sum4/1 -> Abs/1
  Abs/1 -> normalized position/1
  normalized position/1 -> Math Function1/1
  Constant2/1 -> Math Function1/2
  Math Function1/1 -> Gain/1
  Gain/1 -> Math Function/1
  Math Function/1 -> fce [Fmax]/1

== system muscleLegs_task2/Muscle Dynamics/MTU2/CE inverse force-velocity relation ==
  note: CE Inverse Force-Velocity Relationship
  Fv[Fmax] : Inport
  1 : Product  Inputs=/*
  Constant{1,3..4,8} (4 alike) : Constant
  Constant2 : Constant  Value=N
  Constant5 : Constant  Value=N
  Curvature : Gain  Gain=K  SaturateOnIntegerOverflow=on  OutDataTypeStr=Inherit: Same as input  ParamDataTypeStr=Inherit: Same as input
  Curvature1 : Gain  Gain=7.56*K  SaturateOnIntegerOverflow=on  OutDataTypeStr=Inherit: Same as input  ParamDataTypeStr=Inherit: Same as input
  Mux : Mux  Inputs=2
  Mux1 : Mux  Inputs=3
  Mux2 : Mux  Inputs=3
  Slope : Gain  Gain=1e-2  SaturateOnIntegerOverflow=on  OutDataTypeStr=Inherit: Same as input  ParamDataTypeStr=Inherit: Same as input
  Sum1 : Sum  Inputs=|++  InputSameDT=on  SaturateOnIntegerOverflow=on  OutDataTypeStr=Inherit: Same as first input
  Sum2 : Sum  InputSameDT=on  SaturateOnIntegerOverflow=on  OutDataTypeStr=Inherit: Same as first input
  Sum3 : Sum  Inputs=++|  InputSameDT=on  SaturateOnIntegerOverflow=on  OutDataTypeStr=Inherit: Same as first input
  Sum4 : Sum  Inputs=|+-  InputSameDT=on  SaturateOnIntegerOverflow=on  OutDataTypeStr=Inherit: Same as first input
  Sum5 : Sum  Inputs=|-+  InputSameDT=on  SaturateOnIntegerOverflow=on  OutDataTypeStr=Inherit: Same as first input
  Sum6 : Sum  Inputs=-+|  InputSameDT=on  SaturateOnIntegerOverflow=on  OutDataTypeStr=Inherit: Same as first input
  Sum7 : Sum  Inputs=|++  InputSameDT=on  SaturateOnIntegerOverflow=on  OutDataTypeStr=Inherit: Same as first input
  Sum8 : Sum  Inputs=+-|  InputSameDT=on  SaturateOnIntegerOverflow=on  OutDataTypeStr=Inherit: Same as first input
  Sum9 : Sum  InputSameDT=on  SaturateOnIntegerOverflow=on  OutDataTypeStr=Inherit: Same as first input
  concentric branch : Fcn  Expr=u(1) * (u(2)<=1)
  excentric branch : Fcn  Expr=u(2) * (u(1)>1)*(u(1)<=u(3))
  excentric overshoot : Fcn  Expr=u(3) * (u(2)>u(1))
  v_concentric : Product  Inputs=*/
  v_excentric <N : Product  Inputs=*/
  v[vmax] : Outport  VectorParamsAs1DForOutWhenUnconnected=off
  wires:
  Curvature/1 -> Sum3/2
  Constant1/1 -> Sum4/2, Sum3/1
  Sum4/1 -> v_concentric/1
  Sum3/1 -> v_concentric/2
  1/1 -> Sum7/1, Curvature1/1
  Constant4/1 -> Sum7/2, Sum8/1
  Curvature1/1 -> Sum8/2
  Sum8/1 -> v_excentric <N/2
  Sum7/1 -> v_excentric <N/1
  v_concentric/1 -> Mux/1
  Fv[Fmax]/1 -> Sum4/1, Curvature/1, Sum6/2, Mux/2, Mux1/1, Mux2/2
  Sum9/1 -> v[vmax]/1
  Sum2/1 -> Sum9/2
  excentric overshoot/1 -> Sum2/2
  Slope/1 -> Sum1/1
  Constant8/1 -> Sum1/2
  Sum6/1 -> 1/2, Slope/1
  Constant2/1 -> Sum6/1, Sum5/2
  Sum5/1 -> 1/1
  Constant3/1 -> Sum5/1
  Mux/1 -> concentric branch/1
  Mux1/1 -> excentric branch/1
  v_excentric <N/1 -> Mux1/2
  Mux2/1 -> excentric overshoot/1
  concentric branch/1 -> Sum9/1
  excentric branch/1 -> Sum2/1
  Constant5/1 -> Mux1/3, Mux2/1
  Sum1/1 -> Mux2/3

== system muscleLegs_task2/Muscle Dynamics/MTU2/PE force-length relation ==
  note: Parallel Elasticity PE
  lce [lopt] : Inport
  Constant3 : Constant
  Math Function2 : Math  Operator=square  SignedPower=on
  Mux : Mux  Inputs=2
  Sum1 : Sum  Inputs=|+-  InputSameDT=on  SaturateOnIntegerOverflow=on  OutDataTypeStr=Inherit: Same as first input
  force above slack length : Fcn  Expr=u(2) * (u(1)>1)
  reference strain [lopt] : Constant  Value=w_pe
  relative strain : Product  Inputs=*/
  fpe [Fmax] : Outport  VectorParamsAs1DForOutWhenUnconnected=off
  wires:
  Mux/1 -> force above slack length/1
  lce [lopt]/1 -> Mux/1, Sum1/1
  Constant3/1 -> Sum1/2
  Sum1/1 -> relative strain/1
  reference strain [lopt]/1 -> relative strain/2
  relative strain/1 -> Math Function2/1
  Math Function2/1 -> Mux/2
  force above slack length/1 -> fpe [Fmax]/1

== system muscleLegs_task2/Muscle Dynamics/MTU2/SE force-length relation ==
  note: SE Force-Length Relationship
  lse [lslack] : Inport
  eref [lslack] : Inport  Port=2
  Constant1 : Constant
  Math Function : Math  Operator=square  SignedPower=on
  Mux : Mux  Inputs=2
  Sum4 : Sum  Inputs=|+-  InputSameDT=on  SaturateOnIntegerOverflow=on  OutDataTypeStr=Inherit: Same as first input
  force above slack length : Fcn  Expr=u(2)*(u(1)>1)
  relative strain : Product  Inputs=*/
  fse [Fmax] : Outport  VectorParamsAs1DForOutWhenUnconnected=off
  wires:
  Mux/1 -> force above slack length/1
  force above slack length/1 -> fse [Fmax]/1
  Math Function/1 -> Mux/2
  lse [lslack]/1 -> Mux/1, Sum4/1
  relative strain/1 -> Math Function/1
  eref [lslack]/1 -> relative strain/2
  Sum4/1 -> relative strain/1
  Constant1/1 -> Sum4/2

== system muscleLegs_task2/Muscle Dynamics/MTU3/BE force-length relation ==
  note: Buffer Elasticity BE
  lce [lopt] : Inport
  Constant1 : Constant  Value=1-w
  Math Function : Math  Operator=square  SignedPower=on
  Mux1 : Mux  Inputs=2
  Sum4 : Sum  Inputs=|+-  InputSameDT=on  SaturateOnIntegerOverflow=on  OutDataTypeStr=Inherit: Same as first input
  force above slack length : Fcn  Expr=u(2)*(u(1)<0)
  reference strain [lslack] : Constant  Value=w/2
  relative strain : Product  Inputs=*/
  fbe [Fmax] : Outport  VectorParamsAs1DForOutWhenUnconnected=off
  wires:
  lce [lopt]/1 -> Sum4/1
  Mux1/1 -> force above slack length/1
  force above slack length/1 -> fbe [Fmax]/1
  Math Function/1 -> Mux1/2
  relative strain/1 -> Math Function/1
  reference strain [lslack]/1 -> relative strain/2
  Sum4/1 -> relative strain/1, Mux1/1
  Constant1/1 -> Sum4/2

== system muscleLegs_task2/Muscle Dynamics/MTU3/CE force-length relation ==
  note: CE Force-Length Relationship
  lce [lopt] : Inport
  Abs : Abs  SaturateOnIntegerOverflow=off
  Constant1 : Constant
  Constant2 : Constant  Value=3
  Gain : Gain  Gain=log(c)
  Math Function : Math  SignedPower=on
  Math Function1 : Math  Operator=pow  SignedPower=on
  Sum4 : Sum  Inputs=|+-  InputSameDT=on  SaturateOnIntegerOverflow=on  OutDataTypeStr=Inherit: Same as first input
  normalized position : Product  Inputs=*/
  relative width : Constant  Value=w
  fce [Fmax] : Outport  VectorParamsAs1DForOutWhenUnconnected=off
  wires:
  lce [lopt]/1 -> Sum4/1
  relative width/1 -> normalized position/2
  Constant1/1 -> Sum4/2
  Sum4/1 -> Abs/1
  Abs/1 -> normalized position/1
  normalized position/1 -> Math Function1/1
  Constant2/1 -> Math Function1/2
  Math Function1/1 -> Gain/1
  Gain/1 -> Math Function/1
  Math Function/1 -> fce [Fmax]/1

== system muscleLegs_task2/Muscle Dynamics/MTU3/CE inverse force-velocity relation ==
  note: CE Inverse Force-Velocity Relationship
  Fv[Fmax] : Inport
  1 : Product  Inputs=/*
  Constant{1,3..4,8} (4 alike) : Constant
  Constant2 : Constant  Value=N
  Constant5 : Constant  Value=N
  Curvature : Gain  Gain=K  SaturateOnIntegerOverflow=on  OutDataTypeStr=Inherit: Same as input  ParamDataTypeStr=Inherit: Same as input
  Curvature1 : Gain  Gain=7.56*K  SaturateOnIntegerOverflow=on  OutDataTypeStr=Inherit: Same as input  ParamDataTypeStr=Inherit: Same as input
  Mux : Mux  Inputs=2
  Mux1 : Mux  Inputs=3
  Mux2 : Mux  Inputs=3
  Slope : Gain  Gain=1e-2  SaturateOnIntegerOverflow=on  OutDataTypeStr=Inherit: Same as input  ParamDataTypeStr=Inherit: Same as input
  Sum1 : Sum  Inputs=|++  InputSameDT=on  SaturateOnIntegerOverflow=on  OutDataTypeStr=Inherit: Same as first input
  Sum2 : Sum  InputSameDT=on  SaturateOnIntegerOverflow=on  OutDataTypeStr=Inherit: Same as first input
  Sum3 : Sum  Inputs=++|  InputSameDT=on  SaturateOnIntegerOverflow=on  OutDataTypeStr=Inherit: Same as first input
  Sum4 : Sum  Inputs=|+-  InputSameDT=on  SaturateOnIntegerOverflow=on  OutDataTypeStr=Inherit: Same as first input
  Sum5 : Sum  Inputs=|-+  InputSameDT=on  SaturateOnIntegerOverflow=on  OutDataTypeStr=Inherit: Same as first input
  Sum6 : Sum  Inputs=-+|  InputSameDT=on  SaturateOnIntegerOverflow=on  OutDataTypeStr=Inherit: Same as first input
  Sum7 : Sum  Inputs=|++  InputSameDT=on  SaturateOnIntegerOverflow=on  OutDataTypeStr=Inherit: Same as first input
  Sum8 : Sum  Inputs=+-|  InputSameDT=on  SaturateOnIntegerOverflow=on  OutDataTypeStr=Inherit: Same as first input
  Sum9 : Sum  InputSameDT=on  SaturateOnIntegerOverflow=on  OutDataTypeStr=Inherit: Same as first input
  concentric branch : Fcn  Expr=u(1) * (u(2)<=1)
  excentric branch : Fcn  Expr=u(2) * (u(1)>1)*(u(1)<=u(3))
  excentric overshoot : Fcn  Expr=u(3) * (u(2)>u(1))
  v_concentric : Product  Inputs=*/
  v_excentric <N : Product  Inputs=*/
  v[vmax] : Outport  VectorParamsAs1DForOutWhenUnconnected=off
  wires:
  Curvature/1 -> Sum3/2
  Constant1/1 -> Sum4/2, Sum3/1
  Sum4/1 -> v_concentric/1
  Sum3/1 -> v_concentric/2
  1/1 -> Sum7/1, Curvature1/1
  Constant4/1 -> Sum7/2, Sum8/1
  Curvature1/1 -> Sum8/2
  Sum8/1 -> v_excentric <N/2
  Sum7/1 -> v_excentric <N/1
  v_concentric/1 -> Mux/1
  Fv[Fmax]/1 -> Sum4/1, Curvature/1, Sum6/2, Mux/2, Mux1/1, Mux2/2
  Sum9/1 -> v[vmax]/1
  Sum2/1 -> Sum9/2
  excentric overshoot/1 -> Sum2/2
  Slope/1 -> Sum1/1
  Constant8/1 -> Sum1/2
  Sum6/1 -> 1/2, Slope/1
  Constant2/1 -> Sum6/1, Sum5/2
  Sum5/1 -> 1/1
  Constant3/1 -> Sum5/1
  Mux/1 -> concentric branch/1
  Mux1/1 -> excentric branch/1
  v_excentric <N/1 -> Mux1/2
  Mux2/1 -> excentric overshoot/1
  concentric branch/1 -> Sum9/1
  excentric branch/1 -> Sum2/1
  Constant5/1 -> Mux1/3, Mux2/1
  Sum1/1 -> Mux2/3

== system muscleLegs_task2/Muscle Dynamics/MTU3/PE force-length relation ==
  note: Parallel Elasticity PE
  lce [lopt] : Inport
  Constant3 : Constant
  Math Function2 : Math  Operator=square  SignedPower=on
  Mux : Mux  Inputs=2
  Sum1 : Sum  Inputs=|+-  InputSameDT=on  SaturateOnIntegerOverflow=on  OutDataTypeStr=Inherit: Same as first input
  force above slack length : Fcn  Expr=u(2) * (u(1)>1)
  reference strain [lopt] : Constant  Value=w_pe
  relative strain : Product  Inputs=*/
  fpe [Fmax] : Outport  VectorParamsAs1DForOutWhenUnconnected=off
  wires:
  Mux/1 -> force above slack length/1
  lce [lopt]/1 -> Mux/1, Sum1/1
  Constant3/1 -> Sum1/2
  Sum1/1 -> relative strain/1
  reference strain [lopt]/1 -> relative strain/2
  relative strain/1 -> Math Function2/1
  Math Function2/1 -> Mux/2
  force above slack length/1 -> fpe [Fmax]/1

== system muscleLegs_task2/Muscle Dynamics/MTU3/SE force-length relation ==
  note: SE Force-Length Relationship
  lse [lslack] : Inport
  eref [lslack] : Inport  Port=2
  Constant1 : Constant
  Math Function : Math  Operator=square  SignedPower=on
  Mux : Mux  Inputs=2
  Sum4 : Sum  Inputs=|+-  InputSameDT=on  SaturateOnIntegerOverflow=on  OutDataTypeStr=Inherit: Same as first input
  force above slack length : Fcn  Expr=u(2)*(u(1)>1)
  relative strain : Product  Inputs=*/
  fse [Fmax] : Outport  VectorParamsAs1DForOutWhenUnconnected=off
  wires:
  Mux/1 -> force above slack length/1
  force above slack length/1 -> fse [Fmax]/1
  Math Function/1 -> Mux/2
  lse [lslack]/1 -> Mux/1, Sum4/1
  relative strain/1 -> Math Function/1
  eref [lslack]/1 -> relative strain/2
  Sum4/1 -> relative strain/1
  Constant1/1 -> Sum4/2

== system muscleLegs_task2/Muscle Dynamics/MTU4/BE force-length relation ==
  note: Buffer Elasticity BE
  lce [lopt] : Inport
  Constant1 : Constant  Value=1-w
  Math Function : Math  Operator=square  SignedPower=on
  Mux1 : Mux  Inputs=2
  Sum4 : Sum  Inputs=|+-  InputSameDT=on  SaturateOnIntegerOverflow=on  OutDataTypeStr=Inherit: Same as first input
  force above slack length : Fcn  Expr=u(2)*(u(1)<0)
  reference strain [lslack] : Constant  Value=w/2
  relative strain : Product  Inputs=*/
  fbe [Fmax] : Outport  VectorParamsAs1DForOutWhenUnconnected=off
  wires:
  lce [lopt]/1 -> Sum4/1
  Mux1/1 -> force above slack length/1
  force above slack length/1 -> fbe [Fmax]/1
  Math Function/1 -> Mux1/2
  relative strain/1 -> Math Function/1
  reference strain [lslack]/1 -> relative strain/2
  Sum4/1 -> relative strain/1, Mux1/1
  Constant1/1 -> Sum4/2

== system muscleLegs_task2/Muscle Dynamics/MTU4/CE force-length relation ==
  note: CE Force-Length Relationship
  lce [lopt] : Inport
  Abs : Abs  SaturateOnIntegerOverflow=off
  Constant1 : Constant
  Constant2 : Constant  Value=3
  Gain : Gain  Gain=log(c)
  Math Function : Math  SignedPower=on
  Math Function1 : Math  Operator=pow  SignedPower=on
  Sum4 : Sum  Inputs=|+-  InputSameDT=on  SaturateOnIntegerOverflow=on  OutDataTypeStr=Inherit: Same as first input
  normalized position : Product  Inputs=*/
  relative width : Constant  Value=w
  fce [Fmax] : Outport  VectorParamsAs1DForOutWhenUnconnected=off
  wires:
  lce [lopt]/1 -> Sum4/1
  relative width/1 -> normalized position/2
  Constant1/1 -> Sum4/2
  Sum4/1 -> Abs/1
  Abs/1 -> normalized position/1
  normalized position/1 -> Math Function1/1
  Constant2/1 -> Math Function1/2
  Math Function1/1 -> Gain/1
  Gain/1 -> Math Function/1
  Math Function/1 -> fce [Fmax]/1

== system muscleLegs_task2/Muscle Dynamics/MTU4/CE inverse force-velocity relation ==
  note: CE Inverse Force-Velocity Relationship
  Fv[Fmax] : Inport
  1 : Product  Inputs=/*
  Constant{1,3..4,8} (4 alike) : Constant
  Constant2 : Constant  Value=N
  Constant5 : Constant  Value=N
  Curvature : Gain  Gain=K  SaturateOnIntegerOverflow=on  OutDataTypeStr=Inherit: Same as input  ParamDataTypeStr=Inherit: Same as input
  Curvature1 : Gain  Gain=7.56*K  SaturateOnIntegerOverflow=on  OutDataTypeStr=Inherit: Same as input  ParamDataTypeStr=Inherit: Same as input
  Mux : Mux  Inputs=2
  Mux1 : Mux  Inputs=3
  Mux2 : Mux  Inputs=3
  Slope : Gain  Gain=1e-2  SaturateOnIntegerOverflow=on  OutDataTypeStr=Inherit: Same as input  ParamDataTypeStr=Inherit: Same as input
  Sum1 : Sum  Inputs=|++  InputSameDT=on  SaturateOnIntegerOverflow=on  OutDataTypeStr=Inherit: Same as first input
  Sum2 : Sum  InputSameDT=on  SaturateOnIntegerOverflow=on  OutDataTypeStr=Inherit: Same as first input
  Sum3 : Sum  Inputs=++|  InputSameDT=on  SaturateOnIntegerOverflow=on  OutDataTypeStr=Inherit: Same as first input
  Sum4 : Sum  Inputs=|+-  InputSameDT=on  SaturateOnIntegerOverflow=on  OutDataTypeStr=Inherit: Same as first input
  Sum5 : Sum  Inputs=|-+  InputSameDT=on  SaturateOnIntegerOverflow=on  OutDataTypeStr=Inherit: Same as first input
  Sum6 : Sum  Inputs=-+|  InputSameDT=on  SaturateOnIntegerOverflow=on  OutDataTypeStr=Inherit: Same as first input
  Sum7 : Sum  Inputs=|++  InputSameDT=on  SaturateOnIntegerOverflow=on  OutDataTypeStr=Inherit: Same as first input
  Sum8 : Sum  Inputs=+-|  InputSameDT=on  SaturateOnIntegerOverflow=on  OutDataTypeStr=Inherit: Same as first input
  Sum9 : Sum  InputSameDT=on  SaturateOnIntegerOverflow=on  OutDataTypeStr=Inherit: Same as first input
  concentric branch : Fcn  Expr=u(1) * (u(2)<=1)
  excentric branch : Fcn  Expr=u(2) * (u(1)>1)*(u(1)<=u(3))
  excentric overshoot : Fcn  Expr=u(3) * (u(2)>u(1))
  v_concentric : Product  Inputs=*/
  v_excentric <N : Product  Inputs=*/
  v[vmax] : Outport  VectorParamsAs1DForOutWhenUnconnected=off
  wires:
  Curvature/1 -> Sum3/2
  Constant1/1 -> Sum4/2, Sum3/1
  Sum4/1 -> v_concentric/1
  Sum3/1 -> v_concentric/2
  1/1 -> Sum7/1, Curvature1/1
  Constant4/1 -> Sum7/2, Sum8/1
  Curvature1/1 -> Sum8/2
  Sum8/1 -> v_excentric <N/2
  Sum7/1 -> v_excentric <N/1
  v_concentric/1 -> Mux/1
  Fv[Fmax]/1 -> Sum4/1, Curvature/1, Sum6/2, Mux/2, Mux1/1, Mux2/2
  Sum9/1 -> v[vmax]/1
  Sum2/1 -> Sum9/2
  excentric overshoot/1 -> Sum2/2
  Slope/1 -> Sum1/1
  Constant8/1 -> Sum1/2
  Sum6/1 -> 1/2, Slope/1
  Constant2/1 -> Sum6/1, Sum5/2
  Sum5/1 -> 1/1
  Constant3/1 -> Sum5/1
  Mux/1 -> concentric branch/1
  Mux1/1 -> excentric branch/1
  v_excentric <N/1 -> Mux1/2
  Mux2/1 -> excentric overshoot/1
  concentric branch/1 -> Sum9/1
  excentric branch/1 -> Sum2/1
  Constant5/1 -> Mux1/3, Mux2/1
  Sum1/1 -> Mux2/3

== system muscleLegs_task2/Muscle Dynamics/MTU4/PE force-length relation ==
  note: Parallel Elasticity PE
  lce [lopt] : Inport
  Constant3 : Constant
  Math Function2 : Math  Operator=square  SignedPower=on
  Mux : Mux  Inputs=2
  Sum1 : Sum  Inputs=|+-  InputSameDT=on  SaturateOnIntegerOverflow=on  OutDataTypeStr=Inherit: Same as first input
  force above slack length : Fcn  Expr=u(2) * (u(1)>1)
  reference strain [lopt] : Constant  Value=w_pe
  relative strain : Product  Inputs=*/
  fpe [Fmax] : Outport  VectorParamsAs1DForOutWhenUnconnected=off
  wires:
  Mux/1 -> force above slack length/1
  lce [lopt]/1 -> Mux/1, Sum1/1
  Constant3/1 -> Sum1/2
  Sum1/1 -> relative strain/1
  reference strain [lopt]/1 -> relative strain/2
  relative strain/1 -> Math Function2/1
  Math Function2/1 -> Mux/2
  force above slack length/1 -> fpe [Fmax]/1

== system muscleLegs_task2/Muscle Dynamics/MTU4/SE force-length relation ==
  note: SE Force-Length Relationship
  lse [lslack] : Inport
  eref [lslack] : Inport  Port=2
  Constant1 : Constant
  Math Function : Math  Operator=square  SignedPower=on
  Mux : Mux  Inputs=2
  Sum4 : Sum  Inputs=|+-  InputSameDT=on  SaturateOnIntegerOverflow=on  OutDataTypeStr=Inherit: Same as first input
  force above slack length : Fcn  Expr=u(2)*(u(1)>1)
  relative strain : Product  Inputs=*/
  fse [Fmax] : Outport  VectorParamsAs1DForOutWhenUnconnected=off
  wires:
  Mux/1 -> force above slack length/1
  force above slack length/1 -> fse [Fmax]/1
  Math Function/1 -> Mux/2
  lse [lslack]/1 -> Mux/1, Sum4/1
  relative strain/1 -> Math Function/1
  eref [lslack]/1 -> relative strain/2
  Sum4/1 -> relative strain/1
  Constant1/1 -> Sum4/2

== system muscleLegs_task2/Muscle Dynamics/MTU5/BE force-length relation ==
  note: Buffer Elasticity BE
  lce [lopt] : Inport
  Constant1 : Constant  Value=1-w
  Math Function : Math  Operator=square  SignedPower=on
  Mux1 : Mux  Inputs=2
  Sum4 : Sum  Inputs=|+-  InputSameDT=on  SaturateOnIntegerOverflow=on  OutDataTypeStr=Inherit: Same as first input
  force above slack length : Fcn  Expr=u(2)*(u(1)<0)
  reference strain [lslack] : Constant  Value=w/2
  relative strain : Product  Inputs=*/
  fbe [Fmax] : Outport  VectorParamsAs1DForOutWhenUnconnected=off
  wires:
  lce [lopt]/1 -> Sum4/1
  Mux1/1 -> force above slack length/1
  force above slack length/1 -> fbe [Fmax]/1
  Math Function/1 -> Mux1/2
  relative strain/1 -> Math Function/1
  reference strain [lslack]/1 -> relative strain/2
  Sum4/1 -> relative strain/1, Mux1/1
  Constant1/1 -> Sum4/2

== system muscleLegs_task2/Muscle Dynamics/MTU5/CE force-length relation ==
  note: CE Force-Length Relationship
  lce [lopt] : Inport
  Abs : Abs  SaturateOnIntegerOverflow=off
  Constant1 : Constant
  Constant2 : Constant  Value=3
  Gain : Gain  Gain=log(c)
  Math Function : Math  SignedPower=on
  Math Function1 : Math  Operator=pow  SignedPower=on
  Sum4 : Sum  Inputs=|+-  InputSameDT=on  SaturateOnIntegerOverflow=on  OutDataTypeStr=Inherit: Same as first input
  normalized position : Product  Inputs=*/
  relative width : Constant  Value=w
  fce [Fmax] : Outport  VectorParamsAs1DForOutWhenUnconnected=off
  wires:
  lce [lopt]/1 -> Sum4/1
  relative width/1 -> normalized position/2
  Constant1/1 -> Sum4/2
  Sum4/1 -> Abs/1
  Abs/1 -> normalized position/1
  normalized position/1 -> Math Function1/1
  Constant2/1 -> Math Function1/2
  Math Function1/1 -> Gain/1
  Gain/1 -> Math Function/1
  Math Function/1 -> fce [Fmax]/1
